simulink model "RobotX_TrajectoryPlanning2"  (R2024a)
settings: Solver=ode45  StartTime=0.0  StopTime=14  FixedStep=1e-2  MaxStep=1e-3  MinStep=1e-5  RelTol=1e-3
libraries: simulink x7, aerolibconvert2 x6, matrix_library x2, dspinverses x1, RobotX_Lib x1
settings Model: SimulationMode=accelerator  Creator=margaridaestrela  LastModifiedBy=margaridaestrela
settings SolverCC: MaxOrder=2  MaxConsecutiveMinStep=5  ZeroCrossControl=DisableAll  ZeroCrossAlgorithm=Adaptive  MinimalZcImpactIntegration=on  EnableFixedStepZeroCrossing=on  MaxZcPerStep=100
settings DataIOCC: SaveOutput=off  SignalLogging=off  DSMLogging=off  SaveTime=off  ReturnWorkspaceOutputs=off
settings DebuggingCC: SignalInfNanChecking=error

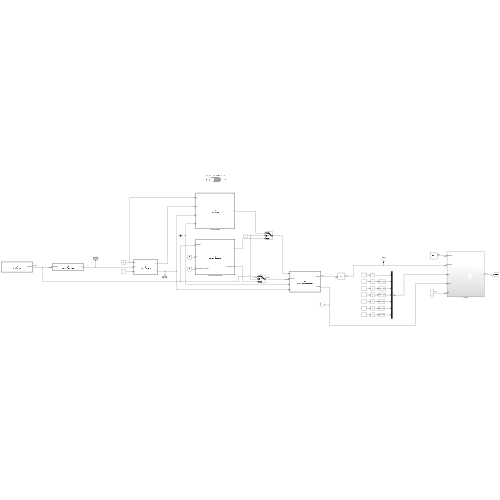
[thumbnail: Simulink's stored preview of the top-level diagram]
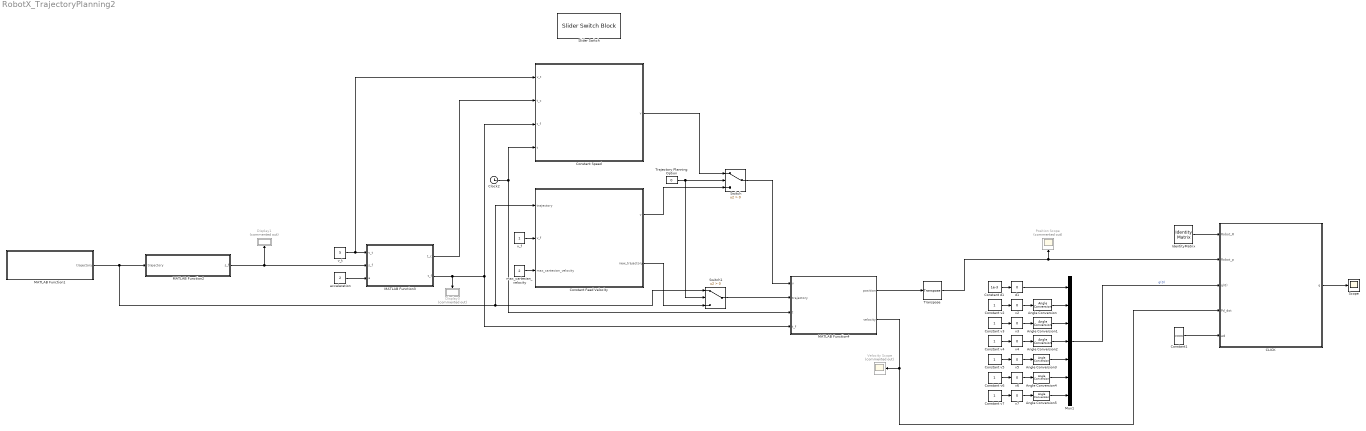
== system RobotX_TrajectoryPlanning2 ==
  Angle Conversion{,1..5} (6 alike) : aerolibconvert2/Angle Conversion  IU=deg  OU=rad
  CLICK : Subsystem
  Clock2 : Clock
  Constant Feed Velocity : MATLAB Function  TreatAsAtomicUnit=on
  Constant Speed : MATLAB Function  TreatAsAtomicUnit=on
  Constant d1 : Constant  Value=1e-3
  Constant v{2..7} (6 alike) : Constant
  Constant1 : Constant  Value=[0;0;0]  VectorParams1D=off
  Display1 : Display  Commented=on
  Display3 : Display  Commented=on
  IdentityMatrix : IdentityMatrix  OutputDimensions=3
  MATLAB Function1 : MATLAB Function  TreatAsAtomicUnit=on
  MATLAB Function2 : MATLAB Function  TreatAsAtomicUnit=on
  MATLAB Function3 : MATLAB Function  TreatAsAtomicUnit=on
  MATLAB Function4 : MATLAB Function  TreatAsAtomicUnit=on
  Mux1 : Mux  Inputs=7
  Position Scope : Scope  Commented=on
  Scope : Scope
  Slider Switch : SliderSwitchBlock
      settings: Values={{'Off', 'On'}, [0 1]}
  Switch : Switch  Criteria=u2 > Threshold  SaturateOnIntegerOverflow=off  InputSameDT=off
  Switch1 : Switch  Criteria=u2 > Threshold  SaturateOnIntegerOverflow=off  InputSameDT=off
  Trajectory Planning Option : Constant  Value=0
  Transpose : matrix_library/Transpose
  Velocity Scope : Scope  Commented=on
  acceleration : Constant  Value=2
  d1 : simulink/Math Operations/Slider Gain  gain=0  low=-350  high=350
  max_cartesian_velocity : Constant  Value=2
  v2 : simulink/Math Operations/Slider Gain  gain=0  low=-170  high=170
  v3 : simulink/Math Operations/Slider Gain  gain=0  low=-190  high=45
  v4 : simulink/Math Operations/Slider Gain  gain=0  low=-120  high=156
  v5 : simulink/Math Operations/Slider Gain  gain=0  low=-185  high=185
  v6 : simulink/Math Operations/Slider Gain  gain=0  low=-120  high=120
  v7 : simulink/Math Operations/Slider Gain  gain=0  low=-350  high=350
  v_f : Constant
  v_t : Constant  Value=5
  wires:
  MATLAB Function2/1(s_f) -> Display1/1, MATLAB Function3/2(s_f)
  v_t/1 -> MATLAB Function3/1(v_t), Constant Speed/1(v_t)
  acceleration/1 -> MATLAB Function3/3(a)
  MATLAB Function3/2(t_f) -> Display3/1, Constant Speed/3(t_f), MATLAB Function4/4(t_f)
  MATLAB Function1/1(trajectory) -> MATLAB Function2/1(trajectory), Constant Feed Velocity/1(trajectory), Switch1/1
  MATLAB Function3/1(t_c) -> Constant Speed/2(t_c)
  Clock2/1 -> MATLAB Function4/3(t), Constant Speed/4(t)
  Constant Speed/1(v) -> Switch/1
  MATLAB Function4/1(position) -> Transpose/1
  Constant v5/1 -> v5/1
  v4/1 -> Angle Conversion2/1
  Mux1/1 -> CLICK/3(q(0))  "q(0)"
  Constant d1/1 -> d1/1
  Constant v4/1 -> v4/1
  Constant1/1 -> CLICK/5(wd)
  Angle Conversion/1 -> Mux1/2
  Angle Conversion4/1 -> Mux1/6
  Constant v6/1 -> v6/1
  Transpose/1 -> CLICK/2(Robot_p), Position Scope/1
  Constant v2/1 -> v2/1
  CLICK/1(q) -> Scope/1
  v7/1 -> Angle Conversion5/1
  v6/1 -> Angle Conversion4/1
  d1/1 -> Mux1/1
  IdentityMatrix/1 -> CLICK/1(Robot_R)
  Constant v3/1 -> v3/1
  Angle Conversion3/1 -> Mux1/5
  v2/1 -> Angle Conversion/1
  Angle Conversion1/1 -> Mux1/3
  Angle Conversion2/1 -> Mux1/4
  Angle Conversion5/1 -> Mux1/7
  v3/1 -> Angle Conversion1/1
  v5/1 -> Angle Conversion3/1
  Constant v7/1 -> v7/1
  MATLAB Function4/2(velocity) -> Velocity Scope/1, CLICK/4(Pd_dot)
  Trajectory Planning Option/1 -> Switch/2, Switch1/2
  Switch/1 -> MATLAB Function4/1(v)
  max_cartesian_velocity/1 -> Constant Feed Velocity/3(max_cartesian_velocity)
  v_f/1 -> Constant Feed Velocity/2(v_f)
  Switch1/1 -> MATLAB Function4/2(trajectory)
  Constant Feed Velocity/2(new_trajectory) -> Switch1/3
  Constant Feed Velocity/1(v) -> Switch/3

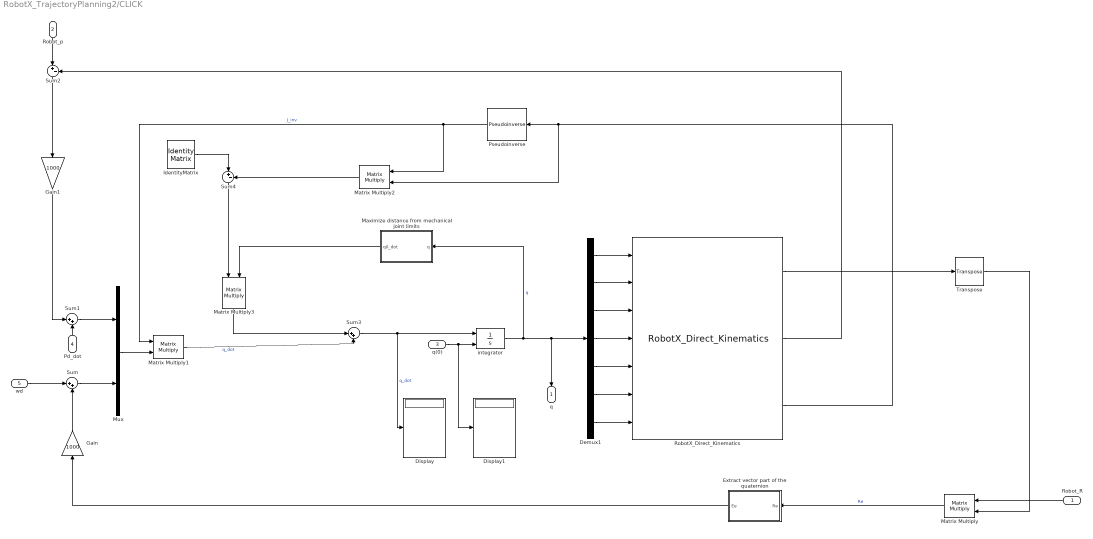
== system RobotX_TrajectoryPlanning2/CLICK ==
  Robot_R : Inport
  Robot_p : Inport  Port=2
  q(0) : Inport  Port=3
  Pd_dot : Inport  Port=4
  wd : Inport  Port=5
  Demux1 : Demux  Outputs=7
  Display : Display
  Display1 : Display
  Extract vector part of the quaternion : MATLAB Function  TreatAsAtomicUnit=on
  Gain : Gain  Gain=1000
  Gain1 : Gain  Gain=1000
  IdentityMatrix : IdentityMatrix  OutputDimensions=7
  Matrix Multiply{,1..3} (4 alike) : Product  Multiplication=Matrix(*)
  Maximize distance from mechanical joint limits : MATLAB Function  TreatAsAtomicUnit=on
  Mux : Mux  Inputs=2
  Pseudoinverse : dspinverses/Pseudoinverse  wanterr=off  SimulateUsing=Interpreted execution
  RobotX_Direct_Kinematics : RobotX_Lib/RobotX_Direct_Kinematics  SystemSampleTime=-1  VariantActivationTime=update diagram  AllowFlexibleInterface=on  Latency=0  AutoFrameSizeCalculation=off
  Sum : Sum  Inputs=|++
  Sum1 : Sum  Inputs=|++
  Sum2 : Sum  Inputs=|+-
  Sum3 : Sum  Inputs=|++
  Sum4 : Sum  Inputs=|+-
  Transpose : matrix_library/Transpose
  integrator : Integrator  InitialConditionSource=external
  q : Outport
  wires:
  Robot_p/1 -> Sum2/1
  Robot_R/1 -> Matrix Multiply/1
  Sum1/1 -> Mux/1
  Matrix Multiply3/1 -> Sum3/1
  Demux1/4 -> RobotX_Direct_Kinematics/4
  Mux/1 -> Matrix Multiply1/2
  Sum/1 -> Mux/2
  Transpose/1 -> Matrix Multiply/2
  Demux1/7 -> RobotX_Direct_Kinematics/7
  Matrix Multiply1/1 -> Sum3/2  "q_dot"
  Pseudoinverse/1 -> Matrix Multiply1/1, Matrix Multiply2/1  "J_inv"
  IdentityMatrix/1 -> Sum4/1
  Gain1/1 -> Sum1/1
  integrator/1 -> Maximize distance from mechanical joint limits/1(q), Demux1/1, q/1  "q"
  Demux1/6 -> RobotX_Direct_Kinematics/6
  RobotX_Direct_Kinematics/3 -> Matrix Multiply2/2, Pseudoinverse/1
  Matrix Multiply/1 -> Extract vector part of the quaternion/1(Re)  "Re"
  Sum2/1 -> Gain1/1
  Demux1/2 -> RobotX_Direct_Kinematics/2
  Demux1/5 -> RobotX_Direct_Kinematics/5
  Maximize distance from mechanical joint limits/1(q0_dot) -> Matrix Multiply3/2
  Demux1/3 -> RobotX_Direct_Kinematics/3
  Matrix Multiply2/1 -> Sum4/2
  Sum3/1 -> Display/1, integrator/1  "q_dot"
  q(0)/1 -> Display1/1, integrator/2
  RobotX_Direct_Kinematics/1 -> Transpose/1
  Gain/1 -> Sum/2
  Demux1/1 -> RobotX_Direct_Kinematics/1
  Sum4/1 -> Matrix Multiply3/1
  RobotX_Direct_Kinematics/2 -> Sum2/2
  Extract vector part of the quaternion/1(Ee) -> Gain/1
  Pd_dot/1 -> Sum1/2
  wd/1 -> Sum/1

== matlab function RobotX_TrajectoryPlanning2/MATLAB Function4 ==
  data: v input; trajectory input; t input; position output; velocity output; t_f input
function [position, velocity] = interpolatePositionVelocity(v, trajectory, t, t_f)
    % Normalize time
    normalized_t = t / t_f;
    
    % Interpolate position
    position = interp1(linspace(0, 1, size(trajectory, 1)), trajectory, normalized_t, 'linear');
    
    % Interpolate velocity
    if size(v, 1) >= 2 % Check if there are at least two data points for interpolation
        velocity = interp1(linspace(0, 1, size(v, 1)), v, normalized_t, 'linear');
    else
        % Handle case where there's only one data point for interpolation
        velocity = v(1, :);
    end
end

== matlab function RobotX_TrajectoryPlanning2/CLICK/Extract vector part of the quaternion ==
  data: Re input; Ee output
function Ee = fcn(Re)
    Ee = zeros(3, 1);
    trace = Re(1,1) + Re(2,2) + Re(3,3);
    if ((trace-1)/2 >= -1 && (trace-1)/2 <= 1)
        v = acos((trace-1)/2);
        if sin(v) ~= 0
            rx = Re(3, 2) - Re(2, 3);
            ry = Re(1, 3) - Re(3, 1);
            rz = Re(2, 1) - Re(1, 2);
    
            Ee = 1/(2*sin(v)) * [rx; ry; rz] * v;
        end
    end
end

== matlab function RobotX_TrajectoryPlanning2/Constant Speed ==
  data: v_t input; t_c input; t_f input; t input; v output
function v = constantSpeed(v_t, t_c, t_f, t)
    v = zeros(size(t));
    acceleration_phase = t < t_c;
    constant_speed_phase = (t >= t_c) & (t <= (t_f - t_c));
    deceleration_phase = (t > (t_f - t_c)) & (t <= t_f);

    v(acceleration_phase) = (v_t / t_c) * t(acceleration_phase);
    v(constant_speed_phase) = v_t;
    v(deceleration_phase) = v_t - (v_t / t_c) * (t(deceleration_phase) - (t_f - t_c));
end

== matlab function RobotX_TrajectoryPlanning2/MATLAB Function1 ==
  data: trajectory output
function trajectory = loadTrajectory()
    data = load('trajectoryData.mat');
    trajectory2D = data.trajectory;

    % Add a Z-coordinate of 0 to each point
    trajectory = [zeros(size(trajectory2D, 1), 1), trajectory2D];
end

== matlab function RobotX_TrajectoryPlanning2/MATLAB Function2 ==
  data: trajectory input; s_f output
function s_f = calculateTotalLength(trajectory)
    % Compute the distance between consecutive points
    diffs = diff(trajectory, 1, 1).^2;
    distances = sqrt(sum(diffs, 2));
    
    % Compute the total length
    s_f = sum(distances);
end

== matlab function RobotX_TrajectoryPlanning2/MATLAB Function3 ==
  data: v_t input; t_c output; s_f input; t_f output; a input
function [t_c, t_f] = calculateTotalTime(v_t, s_f, a)
    % Calculate time to reach maximum velocity (acceleration phase)
    t_c = v_t / a;
    
    % Calculate distance covered during acceleration (and deceleration)
    d_c = 0.5 * a * t_c^2;
    
    % Calculate distance covered at constant velocity
    d_const = s_f - 2 * d_c;
    
    % Check if the distance for acceleration and deceleration is feasible
    if d_c * 2 > s_f
        error('Total distance is too short for the given acceleration and maximum velocity.');
    end
    
    % Calculate time for constant velocity phase
    t_const = d_const / v_t;
    
    % Total time of the trajectory
    t_f = t_c + t_const + t_c; % t_c is used for both acceleration and deceleration phases
end

== matlab function RobotX_TrajectoryPlanning2/CLICK/Maximize distance from mechanical joint limits ==
  data: q0_dot output; q input
function q0_dot = fcn(q)
    n = size(q, 1);

    q_max = max(q);
    q_min = min(q);
    epsilon = 1e-6; % A small value to prevent division by zero
    q_dif = q_max - q_min + epsilon;

    % Manually derive the differentiation
    w_diff = - (q - q_max)/(n * q_dif^2);
    q0_dot = 2 * w_diff;
end

== matlab function RobotX_TrajectoryPlanning2/Constant Feed Velocity ==
  data: v output; trajectory input; v_f input; max_cartesian_velocity input; new_trajectory output
function [v, new_trajectory] = constantFeedVelocity(trajectory, v_f, max_cartesian_velocity)
    % Calculate distances between consecutive points in the trajectory
    distances = sqrt(sum(diff(trajectory).^2, 2));
    
    % Calculate the time intervals required to travel each segment at the feed velocity
    time_intervals = distances / v_f;
    
    % Initialize positions and velocities
    n_points = size(trajectory, 1);
    new_trajectory = trajectory;
    v = zeros(n_points, 1);
    
    % Calculate velocities ensuring max cartesian velocity constraint
    for i = 1:n_points-1
        current_distance = distances(i);
        required_time = time_intervals(i) + 1e-6;
        v(i) = current_distance / required_time;
        
        % Ensure velocity does not exceed max cartesian velocity
        if v(i) > max_cartesian_velocity
            v(i) = max_cartesian_velocity;
        end
        
        % Adjust the position based on the velocity
        if i > 1
            new_trajectory(i+1, :) = new_trajectory(i, :) + (v(i) / v_f) * (trajectory(i+1, :) - trajectory(i, :));
        end
    end
    
    % Handle the last point
    v(end) = v(end-1);
end
